simulink library "galipeur_lib"  (R2017a)
settings: Solver=VariableStepAuto  StartTime=0.0  StopTime=10.0  RelTol=1e-3
settings Model: Creator=jdam  LastModifiedBy=jdam

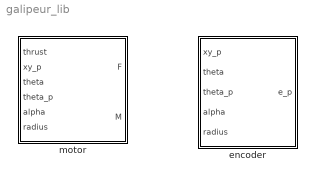
== system galipeur_lib ==
  encoder : Subsystem
  motor : Subsystem

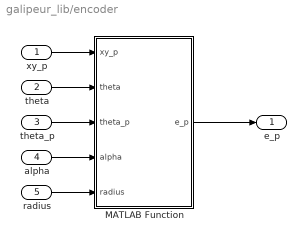
== system galipeur_lib/encoder ==
  xy_p : Inport
  theta : Inport  Port=2
  theta_p : Inport  Port=3
  alpha : Inport  Port=4
  radius : Inport  Port=5
  MATLAB Function : MATLAB Function  TreatAsAtomicUnit=on
  e_p : Outport
  wires:
  xy_p/1 -> MATLAB Function/1(xy_p)
  theta/1 -> MATLAB Function/2(theta)
  theta_p/1 -> MATLAB Function/3(theta_p)
  alpha/1 -> MATLAB Function/4(alpha)
  radius/1 -> MATLAB Function/5(radius)
  MATLAB Function/1(e_p) -> e_p/1

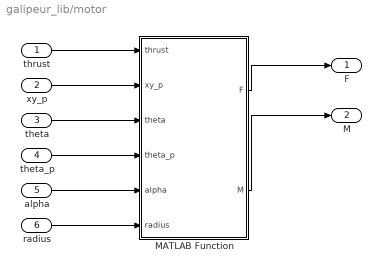
== system galipeur_lib/motor ==
  thrust : Inport
  xy_p : Inport  Port=2
  theta : Inport  Port=3
  theta_p : Inport  Port=4
  alpha : Inport  Port=5
  radius : Inport  Port=6
  MATLAB Function : MATLAB Function  TreatAsAtomicUnit=on
  F : Outport
  M : Outport  Port=2
  wires:
  thrust/1 -> MATLAB Function/1(thrust)
  xy_p/1 -> MATLAB Function/2(xy_p)
  theta/1 -> MATLAB Function/3(theta)
  theta_p/1 -> MATLAB Function/4(theta_p)
  alpha/1 -> MATLAB Function/5(alpha)
  radius/1 -> MATLAB Function/6(radius)
  MATLAB Function/1(F) -> F/1
  MATLAB Function/2(M) -> M/1

== matlab function galipeur_lib/encoder/MATLAB Function ==
  data: xy_p input; e_p output; theta input; theta_p input; alpha input; radius input
function e_p = fcn(xy_p,theta,theta_p,alpha,radius)
% xy_p: robot velocity in ground reference (xp, yp)
% alpha: motor orientation placement relative to robot
% radius: motor distance from robot CG relative to robot
% theta: robot orientation relative to ground
% theta_p: robot rotation speed

% compute unitary vector perpendicular to thrust
up = [cos(theta+alpha); sin(theta+alpha)];
% compute unitary vector along thrust
ut = [-sin(theta+alpha); cos(theta+alpha)];

% transport speed to contact point
vm = xy_p + radius*theta_p*ut;

% project speed onto unitary thrust vector
e_p = dot(vm,ut);

== matlab function galipeur_lib/motor/MATLAB Function ==
  data: thrust input; F output; xy_p input; theta input; theta_p input; alpha input; radius input; M output
function [F,M]= fcn(thrust, xy_p, theta, theta_p, alpha, radius)
% thrust: motor thrust in N at contact
% xy_p: robot velocity in ground reference (xp, yp)
% alpha: motor orientation placement relative to robot
% radius: motor distance from robot CG relative to robot
% theta: robot orientation relative to ground
% theta_p: robot rotation speed

% compute unitary vector perpendicular to thrust
up = [cos(theta+alpha); sin(theta+alpha)];
% compute unitary vector along thrust
ut = [-sin(theta+alpha); cos(theta+alpha)];

% transport velocity to contact point
vm = xy_p + radius*theta_p*ut;

% project velocity along thrust (in motor)
vt = dot(vm,ut);
% project velocity perpendicular to thrust (rolling omniwheel)
vp = dot(vm,up);

ft = 0.3;
fp = 0.1;
% compute sum of forces for this motor
F = thrust*ut - ft*vt*ut - fp*vp*up;
% compute momentum at robot CoG 
GM = up*radius;
momentum = cross([GM(1);GM(2);0],[F(1);F(2);0]);
M = momentum(3);
